simulink model "IDC_CYCLE"  (R2023b)
settings: Solver=VariableStepAuto  StartTime=0.0  StopTime=simtime  RelTol=1e-3
values from neighbouring files (symbols this model uses):
  Aera = 2.5    [IDC_CODE.m]    (also in MIDC_CODE.m; WLTP_CODE.m)
  battery_energy = 20    [IDC_CODE.m]    (also in MIDC_CODE.m; WLTP_CODE.m)
  Cd = 0.3    [IDC_CODE.m]    (also in MIDC_CODE.m; WLTP_CODE.m)
  CRR = 10    [IDC_CODE.m]    (also in MIDC_CODE.m; WLTP_CODE.m)
  DOD = 0.9    [IDC_CODE.m]    (also in MIDC_CODE.m; WLTP_CODE.m)
  g = 9.81    [IDC_CODE.m]    (also in MIDC_CODE.m; WLTP_CODE.m)
  Grade = 0    [IDC_CODE.m]    (also in MIDC_CODE.m; WLTP_CODE.m)
  m = 1200    [IDC_CODE.m]    (also in MIDC_CODE.m; WLTP_CODE.m)
  mi = imf * m    (= 1242)    [IDC_CODE.m]    (also in MIDC_CODE.m; WLTP_CODE.m)
  motor_Eff = 0.8    [IDC_CODE.m]    (also in MIDC_CODE.m; WLTP_CODE.m)
  rho = 1.17692    [IDC_CODE.m]    (also in MIDC_CODE.m; WLTP_CODE.m)
  trans_Eff = 0.93    [IDC_CODE.m]    (also in MIDC_CODE.m; WLTP_CODE.m)
libraries: slpidlib x1
settings Model: Creator=howde  LastModifiedBy=howde

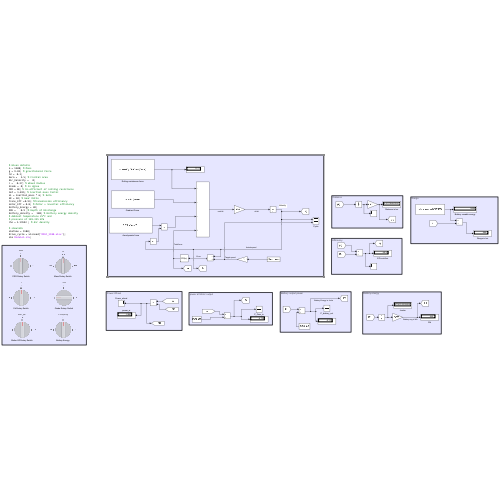
[thumbnail: Simulink's stored preview of the top-level diagram]
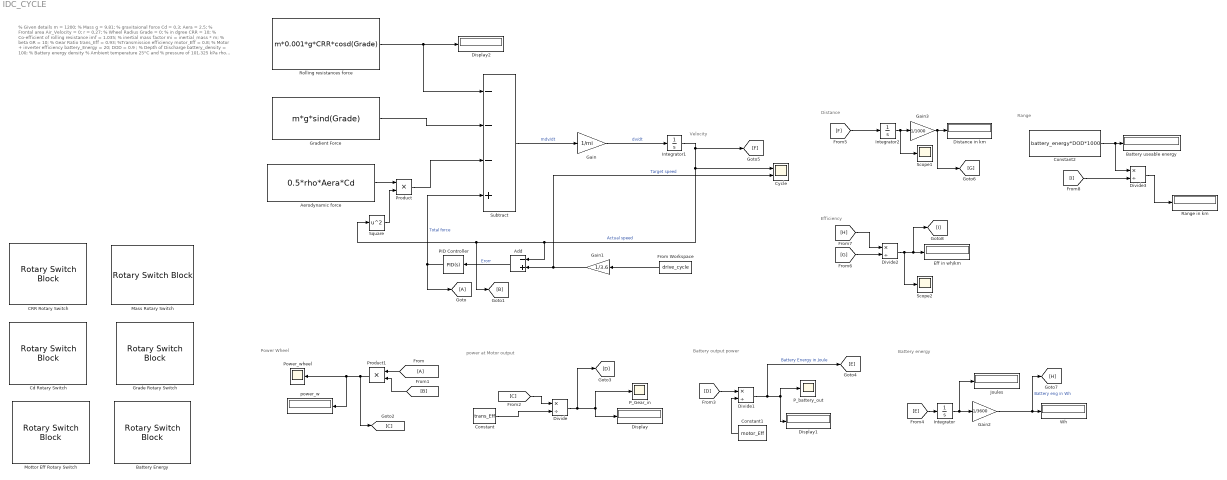
== system IDC_CYCLE ==
  note: Efficiency
  note: Power Wheel
  note: Battery output power
  note: Range
  note: % Given details
      | m = 1200; % Mass
      | g = 9.81; % gravitaional force
      | Cd = 0.3;
      | Aera = 2.5; % Frontal area
      | Air_Velocity = 0;
      | r = 0.27; % Wheel Radius
      | Grade = 0; % in dgree
      | CRR = 10; % Co-efficient of rolling resistance
      | imf = 1.035; % inertial mass factor
      | mi = inertial_mass * m; % beta
      | GR = 10; % Gear Ratio
      | trans_Eff = 0.93; %Transmission efficiency
      | motor_Eff = 0.8; % Motor + inverter efficiency
      | battery_Energy = 20;
      | DOD = 0.9 ; % Depth of Discharge
      | battery_density = 100; % Battery energy density
      | % Ambient temperature 25°C and
      | % pressure of 101.325 kPa
      | rho = 1.17692 ; % Air density
      |
      | % simulnik
      | simtime = 1180;
      | drive_cycle = xlsread( 'MIDC_1180.xlsx' );
      | sim Module1.slx ;
  note: Battery energy
  note: Velocity
  note: Distance
  note: power at Motor output
  Add : Sum  Inputs=-+
  Aerodynamic force : Constant  Value=0.5*rho*Aera*Cd
  Battery Energy : RotarySwitchBlock
      settings: Values={{'15', '20', '25'}, [15 20 25]}
  Battery useable energy : Display
  CRR Rotary Switch : RotarySwitchBlock
      settings: Values={{'8', '10', '12'}, [8 10 12]}
  Cd Rotary Switch : RotarySwitchBlock
      settings: Values={{'0.2', '0.3', '0.4'}, [0.2 0.3 0.4]}
  Constant : Constant  Value=trans_Eff
  Constant1 : Constant  Value=motor_Eff
  Constant2 : Constant  Value=battery_energy*DOD*1000
  Cycle : Scope  NumInputPorts=2
  Display : Display
  Display1 : Display
  Display2 : Display
  Distance in km : Display
  Divide{,1..3} (4 alike) : Product  Inputs=*/
  Eff in wh/km : Display
  From : From
  From Workspace : FromWorkspace  VariableName=drive_cycle
  Gain : Gain  Gain=1/mi
  Gain1 : Gain  Gain=1/3.6
  Gain2 : Gain  Gain=1/3600
  Gain3 : Gain  Gain=1/1000
  Goto : Goto
  Grade Rotary Switch : RotarySwitchBlock
      settings: Values={{'0', '5', '-5'}, [0 5 -5]}
  "Gradient Force " : Constant  Value=m*g*sind(Grade)
  Integrator : Integrator
  Integrator1 : Integrator
  Integrator2 : Integrator
  Joules : Display
  Mass Rotary Switch : RotarySwitchBlock
      settings: Values={{'1000', '1200', '1400'}, [1000 1200 1400]}
  Mottor Eff Rotary Switch : RotarySwitchBlock
      settings: Values={{'0.7', '0.8', '0.9'}, [0.7 0.8 0.9]}
  PID Controller : slpidlib/PID Controller  Controller=PID  Form=Parallel  TimeDomain=Continuous-time  UseExternalTs=off  SampleTime=-1  IntegratorMethod=Forward Euler  FilterMethod=Forward Euler  ControllerParametersSource=internal  P=3600  I=0  UseKiTs=off  D=1  N=100  UseFilter=on  TunerSelectOption=Transfer Function Based (PID Tuner App)  InitialConditionSource=internal  InitialConditionForIntegrator=0  InitialConditionForFilter=0  DifferentiatorICPrevScaledInput=0  ExternalReset=none  TrackingMode=off  Kt=1  LimitOutput=off  SatLimitsSource=internal  UpperSaturationLimit=inf  LowerSaturationLimit=-inf  LinearizeAsGain=on  AntiWindupMode=none  Kb=1  LimitIntegrator=off  UpperIntegratorSaturationLimit=inf  LowerIntegratorSaturationLimit=-inf  POutMin=[]  POutMax=[]  IOutMin=[]  IOutMax=[]  DOutMin=[]  DOutMax=[]  NOutMin=[]  NOutMax=[]  SumOutMin=[]  SumOutMax=[]  SaturationOutMin=[]  SaturationOutMax=[]  PParamMin=[]  PParamMax=[]  IParamMin=[]  IParamMax=[]  DParamMin=[]  DParamMax=[]  NParamMin=[]  NParamMax=[]  KbParamMin=[]  KbParamMax=[]  KtParamMin=[]  KtParamMax=[]  KbOutMin=[]  KbOutMax=[]  KtOutMin=[]  KtOutMax=[]  IntegratorOutMin=[]  IntegratorOutMax=[]  FilterOutMin=[]  FilterOutMax=[]  SumI1OutMin=[]  SumI1OutMax=[]  SumI2OutMin=[]  SumI2OutMax=[]  SumI3OutMin=[]  SumI3OutMax=[]  SumI4OutMin=[]  SumI4OutMax=[]  SumDOutMin=[]  SumDOutMax=[]  DifferentiatorOutMin=[]  DifferentiatorOutMax=[]  FilterDiffOutCoefMin=[]  FilterDiffOutCoefMax=[]  ReciprocalOutMin=[]  ReciprocalOutMax=[]  SumDenOutMin=[]  SumDenOutMax=[]  SumNumOutMin=[]  SumNumOutMax=[]  DivideOutMin=[]  DivideOutMax=[]  UdiffTsProdOutMin=[]  UdiffTsProdOutMax=[]  NTsProdOutMin=[]  NTsProdOutMax=[]  UintegralTsProdOutMin=[]  UintegralTsProdOutMax=[]  UngainTsProdOutMin=[]  UngainTsProdOutMax=[]  ClampingZeroOutDataTypeStr=Inherit: Inherit via back propagation  ClampingZeroOutMin=[]  ClampingZeroOutMax=[]  FilterDenConstantOutDataTypeStr=Inherit: Inherit via back propagation  FilterDenConstantOutMin=[]  FilterDenConstantOutMax=[]  PCopyOutDataTypeStr=Inherit: Inherit via back propagation  PCopyOutMin=[]  PCopyOutMax=[]  NCopyOutDataTypeStr=Inherit: Inherit via back propagation  NCopyOutMin=[]  NCopyOutMax=[]  IntegratorContinuousStateAttributes=''  IntegratorStateMustResolveToSignalObject=off  IntegratorRTWStateStorageClass=Auto  FilterContinuousStateAttributes=''  FilterStateMustResolveToSignalObject=off  FilterRTWStateStorageClass=Auto  ParallelPVariant=InternalParameters  IdealPVariant=Disabled  IVariant=InternalParameters  DVariant=InternalParameters  IntegratorVariant=Continuous  SatVariant=Disabled  AWVariant=Passthrough  PCopyVariant=Disabled  TRVariant=Disabled  FdbkBlocksVariant=Forward  IdealPFdbkVariant=Disabled  SatFdbkVariant=Disabled  DerivativeFilterVariant=ContFilter  NVariant=InternalParameters  NCopyVariant=Disabled  FilterICVariant=InternalICsFilter  IntegratorICVariant=InternalICs  ExternalResetVariant=Disabled  TRSumVariant=Passthrough  SumFdbkVariant=Disabled  SumVariant=Sum_PID  TsampFilterVariant=InternalTs  TsampNgainVariant=Passthrough  TsampIntegralVariant=Disabled_SignalSpec  ExternalSaturationOutDataTypeStr=Inherit: Same as second input
  P_Gear_in : Scope
  P_battery_out : Scope
  Power_wheel : Scope
  Product : Product
  Product1 : Product
  Range in km : Display
  Rolling resistances force : Constant  Value=m*0.001*g*CRR*cosd(Grade)
  Scope1 : Scope
  Scope2 : Scope
  Square : Math  Operator=square
  Subtract : Sum  Inputs=---+
  Wh : Display
  power_w : Display
  wires:
  [C] -> Divide/1
  Square/1 -> Product/2
  PID Controller/1 -> Goto/1, Subtract/4  "Total force"
  Gain1/1 -> Cycle/2, Add/2  "Target speed"
  [H] -> Divide2/1
  Add/1 -> PID Controller/1  "Erorr"
  Aerodynamic force/1 -> Product/1
  [I] -> Divide3/2
  Integrator/1 -> Joules/1, Gain2/1
  Divide1/1 -> [E], Display1/1, P_battery_out/1  "Battery Energy in Joule"
  From Workspace/1 -> Gain1/1
  Constant2/1 -> Divide3/1, Battery useable energy/1
  [B] -> Product1/2
  Gain2/1 -> [H], Wh/1  "Battery eng in Wh"
  Divide3/1 -> Range in km/1
  Rolling resistances force/1 -> Display2/1, Subtract/1
  Integrator2/1 -> Scope1/1, Gain3/1
  Gain3/1 -> [G], Distance in km/1
  Constant/1 -> Divide/2
  Product1/1 -> power_w/1, Power_wheel/1, [C]
  Product/1 -> Subtract/3
  [E] -> Integrator/1
  Subtract/1 -> Gain/1  "mdv/dt"
  From/1 -> Product1/1
  Integrator1/1 -> [F], [B], Square/1, Add/1, Cycle/1  "Actual speed"
  [G] -> Divide2/2
  Gain/1 -> Integrator1/1  "dv/dt"
  [D] -> Divide1/1
  Divide/1 -> [D], Display/1, P_Gear_in/1
  "Gradient Force "/1 -> Subtract/2
  [F] -> Integrator2/1
  Constant1/1 -> Divide1/2
  Divide2/1 -> Scope2/1, [I], Eff in wh/km/1
